simulink library "KL_DeviceData_Hvs"  (Simulink 7.8)
settings: Solver=ode45  StartTime=0.0  StopTime=10.0  RelTol=1e-3
settings Model: Creator=KLJS168  LastModifiedBy=KLJS168

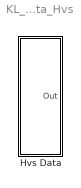
== system KL_DeviceData_Hvs ==
  Hvs Data : Subsystem

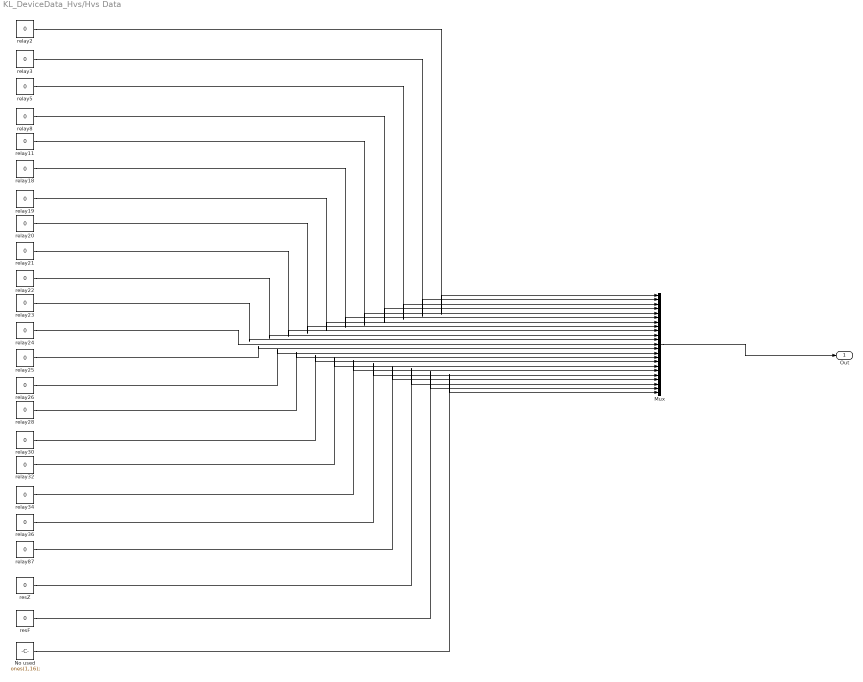
== system KL_DeviceData_Hvs/Hvs Data ==
  Mux : Mux  Inputs=23
  No used : Constant  Value=ones(1,16);
  relay{2..3,5,8,11,18..26,28,30,32,34,36,87} (20 alike) : Constant  Value=0
  resF : Constant  Value=0
  resZ : Constant  Value=0
  Out : Outport
  wires:
  Mux/1 -> Out/1
  No used/1 -> Mux/23
  resF/1 -> Mux/22
  resZ/1 -> Mux/21
  relay87/1 -> Mux/20
  relay36/1 -> Mux/19
  relay34/1 -> Mux/18
  relay32/1 -> Mux/17
  relay30/1 -> Mux/16
  relay28/1 -> Mux/15
  relay26/1 -> Mux/14
  relay25/1 -> Mux/13
  relay24/1 -> Mux/12
  relay23/1 -> Mux/11
  relay22/1 -> Mux/10
  relay21/1 -> Mux/9
  relay20/1 -> Mux/8
  relay19/1 -> Mux/7
  relay18/1 -> Mux/6
  relay11/1 -> Mux/5
  relay8/1 -> Mux/4
  relay5/1 -> Mux/3
  relay3/1 -> Mux/2
  relay2/1 -> Mux/1
